simulink model "MSREPrimaryLoop_PlantLevel"  (R2024a)
settings: Solver=VariableStepAuto  StartTime=0.0  StopTime=500000  MaxStep=0.1  RelTol=1e-3
undefined symbols (not defined in the file): a_f, a_g, axialFuelImportance, axialGraphiteImportance, axialPowerFraction, beta, beta_t, bubbleSaturationLevel, bypassRatio, C0, coolantPHXChannelLength, coolantPHXDh, coolantPHXFlowArea, coreCorrectionNominalFlowRate, coreDowncomerArea, coreDowncomerHydraulicDiameter, coreDowncomerLength, coreDowncomerVolume, coreFlowArea, coreFuelVolume, coreInletFlowDistributerArea, coreInletFlowDistributerHydralicDiameter, coreInletFlowDistributerLength, coreInletFlowDistributerVolume, coreLowerPlenumArea, coreLowerPlenumHydraulicDiameter, coreLowerPlenumLength, coreLowerPlenumVolume, coreUpperPlenumArea, coreUpperPlenumLength, coreUpperPlenumVolume, coreVolume, cpGraphite, day, decayScale, decaySSFraction, dissolusionRatio, dMin, dScale, dsmConst, DXeG, externalReactivity, Fiss_factor, fuelChannelHydrualicDiameter, fuelChannelLength, fuelDepositRatio, fuelFraction, fuelGraphiteArea, fuelGraphiteHeatTransferCoefficient, gamma0, gamma1, gamma2, gasExchangeRatio, gasMixingEfficiency, gasPurgeRate, gasStrippingEfficiency, graphiteKDiff, graphiteUnitCellThickness, initialIodineConcentration, InitialXeMolarConcentration ... (+66)
libraries: fl_lib x291, nesl_utility x101, SimscapeFluids_lib x24, simulink x5, slpidlib x1
(part 13 of 13)

== system MSREPrimaryLoop_PlantLevel/Reactor/CoreTH&Inerti/UpperPlenum/XenonCalc/Salt/Subsystem1 ==
  Gas : Inport
  Add1 : Sum  Inputs=+-
  Constant : Constant
  Subsystem : Subsystem  ReferencedSubsystem=GasToAlpha
  1-alpha : Outport
  wires:
  Gas/1 -> Subsystem/1
  Constant/1 -> Add1/1
  Subsystem/1 -> Add1/2
  Add1/1 -> 1-alpha/1

== system MSREPrimaryLoop_PlantLevel/Reactor/Reactivity&PKE/Reactivity&PKE/REACTIVITY/ExternalReactivity/Constatnt ==
  Constant : Constant  Value=0
  y : Outport
  wires:
  Constant/1 -> y/1

== system MSREPrimaryLoop_PlantLevel/Reactor/Reactivity&PKE/Reactivity&PKE/REACTIVITY/ExternalReactivity/Frequency ==
  Sine Wave : Sin  Amplitude=1e-5  Frequency=testFrequency  SampleTime=0.1
  y : Outport
  wires:
  Sine Wave/1 -> y/1

== system MSREPrimaryLoop_PlantLevel/Reactor/Reactivity&PKE/Reactivity&PKE/REACTIVITY/ExternalReactivity/Step ==
  Step : Step  Time=3*day + 1  After=stepReactivity  SampleTime=0
  y : Outport
  wires:
  Step/1 -> y/1

== system MSREPrimaryLoop_PlantLevel/Reactor/Reactivity&PKE/Reactivity&PKE/REACTIVITY/ExternalReactivity/White Noise ==
  Band-Limited White Noise : simulink/Sources/Band-Limited White Noise  Cov=1e-10  Ts=0.1  seed=[23341]
  y : Outport
  wires:
  Band-Limited White Noise/1 -> y/1

== system MSREPrimaryLoop_PlantLevel/Reactor/CoreTH&Inerti/Core/CoreXenonCalc/InterphaseTranfser/Constitutive/Subsystem ==
  note: Include the form loss to averaged frictional factor as a rough estimate.
  PLoss : Inport
  Dh : Inport  Port=2
  ul : Inport  Port=3
  alpha : Inport  Port=4
  Absolute Reference (TL) : fl_lib/Thermal Liquid/Elements/Absolute Reference (TL)
  Constant : Constant  Value=dissolusionRatio
  Constant1 : Constant  Value=dMin
  Constant2 : Constant  Value=dScale
  Constant3 : Constant  Value=dsmConst
  Divide : Product  Inputs=**//
  Gain : Gain  Gain=2/CoreLength
  MATLAB Function1 : MATLAB Function  TreatAsAtomicUnit=on
  MATLAB Function2 : MATLAB Function  TreatAsAtomicUnit=on
  Math Function : Math  Operator=square
  PS-Simulink Converter : nesl_utility/PS-Simulink Converter  PhysicalDomain=network_engine_domain  SubClassName=ps_output  LeftPortType=input  RightPortType=output  PseudoPeriodic=off  Frequencies=[]  VectorFormat=1-D array  Unit=inherit  AffineConversion=off
  PS-Simulink Converter1 : nesl_utility/PS-Simulink Converter  PhysicalDomain=network_engine_domain  SubClassName=ps_output  LeftPortType=input  RightPortType=output  PseudoPeriodic=off  Frequencies=[]  VectorFormat=1-D array  Unit=inherit  AffineConversion=off
  Pressure & Temperature Sensor (TL) : fl_lib/Thermal Liquid/Sensors/Pressure & Temperature Sensor (TL)  reference=foundation.enum.MeasurementReference.difference  pressure=true  pressure_spec=foundation.enum.PressureMeasementSpec.Absolute  temperature=true
      settings: InternalSimscapePortConfiguration="{\"Bottom\":[{\"id\":\"T\",\"label\":\"T\",\"type\":\"output\"}],\"Left\":[{\"id\":\"A\",\"label\":\"A\",\"type\":\"foundation.thermal_liquid.thermal_liquid\"}],\"Right\":[{\"id\":\"B\",\"label\":\"B\",\"type\":\"foundation.thermal_liquid.thermal_liquid\"},{\"id\":\"P\",\"label\":\"P\",\"type\":\"output\"}],\"Top\":[]}"
  Simscape Component : SimscapeComponentBlock  SourceFile=TL_FullSensor  ComponentPath=TL_FullSensor  ComponentVariants="[\"TL_FullSensor\"]"  ComponentVariantNames="[\"TL_FullSensor\"]"  ClassName=TL_FullSensor  SchemaVersion=1
      settings: CopyFcn=simscape.engine.sli.internal.componentblockcallback(gcbh,'COPY')  PreCopyFcn=simscape.engine.sli.internal.componentblockcallback(gcbh,'PRECOPY')  PreDeleteFcn=simscape.engine.sli.internal.componentblockcallback(gcbh,'PREDELETE')  InternalSimscapePortConfiguration="{\"Bottom\":[],\"Left\":[{\"id\":\"A\",\"label\":\"A\",\"type\":\"foundation.thermal_liquid.thermal_liquid\"}],\"Right\":[{\"id\":\"U\",\"label\":\"u\",\"type\":\"output\"},{\"id\":\"RHO\",\"label\":\"rho\",\"type\":\"output\"},{\"id\":\"CP\",\"label\":\"cp\",\"type\":\"output\"},{\"id\":\"NU\",\"label\":\"nu\",\"type\":\"output\"}],\"Top\":[]}"
      mask Type: Thermodynamic Properties Sensor (TL)
      mask Display: color('red');plot([0 1 1 0 0],[0 0 1 1 0]);plot([0.7,1],[1,0.7]);plot(-2,-1.75);plot(3, 1);disp('\n.ssc\nUnresolved')
  Terminator1 : Terminator
  Ref : PMIOPort  Side=Right
  f_Combined : Outport
  dsm : Outport  Port=2
  wires:
  Dh/1 -> Divide/2, MATLAB Function1/2(D)
  MATLAB Function2/1(sigma) -> MATLAB Function1/5(sigma)
  PS-Simulink Converter1/1 -> MATLAB Function2/1(T)
  ul/1 -> Math Function/1, MATLAB Function1/3(jl)
  PS-Simulink Converter/1 -> Divide/4, MATLAB Function1/4(rhol)
  PLoss/1 -> Gain/1
  Divide/1 -> f_Combined/1, MATLAB Function1/1(f)
  Gain/1 -> Divide/1
  Math Function/1 -> Divide/3
  alpha/1 -> MATLAB Function1/6(alpha)
  Constant/1 -> MATLAB Function1/7(alphaDissolve)
  Constant1/1 -> MATLAB Function1/8(dMin)
  Constant2/1 -> MATLAB Function1/9(scale)
  Constant3/1 -> dsm/1
  MATLAB Function1/1(dsm) -> Terminator1/1
  connections:
  Simscape Component/RConn2 -- PS-Simulink Converter/LConn1
  Simscape Component/LConn1 -- Pressure & Temperature Sensor (TL)/LConn1 -- Ref/RConn1
  Pressure & Temperature Sensor (TL)/RConn3 -- PS-Simulink Converter1/LConn1
  Pressure & Temperature Sensor (TL)/RConn1 -- Absolute Reference (TL)/LConn1

== system MSREPrimaryLoop_PlantLevel/Reactor/CoreTH&Inerti/Core/CoreXenonCalc/InterphaseTranfser/GraphiteInterchangeModel/GasDiffusivityScale ==
  T : Inport
  Constant : Constant  Value=1.5
  Divide : Product  Inputs=*/
  Divide1 : Product  Inputs=*/
  PReff : Constant  Value=1.013e5
  Power : Math  Operator=pow
  Product : Product  Inputs=3
  TRef : Constant  Value=900
  XeReferenceDiff : Constant  Value=DXeG
  DiffGas : Outport
  wires:
  T/1 -> Divide/1
  TRef/1 -> Divide/2
  Divide/1 -> Power/1
  Constant/1 -> Power/2
  PReff/1 -> Divide1/1
  [coreAveragePressure] -> Divide1/2
  Power/1 -> Product/1
  Divide1/1 -> Product/2
  XeReferenceDiff/1 -> Product/3
  Product/1 -> DiffGas/1

== system MSREPrimaryLoop_PlantLevel/Reactor/CoreTH&Inerti/Core/Subsystem2/Subsystem2/If Action Subsystem/SolubilityModificationEqual ==
  note: The idea is that when the dissolved gas comes back out, it is at the same salt concentration, assuming the nucleation process is fast, and it absorbed all xenon at the nucleation site but diffusion is not yet to kick in. As for the absorption into the old bubble, the saturation may be closer to 0, but never the less, the saturation level is already close to zero.
  XeIn : Inport
  CoreGas : Inport  Port=2
  DissolvedGas : Inport  Port=3
  Add : Sum
  Add1 : Sum
  AddedBackGas : Sum
  Constant : Constant
  Demux : Demux  Outputs=2
  Divide : Product  Inputs=**/
  Divide1 : Product  Inputs=*/
  Mux : Mux  Inputs=2
  XeOut : Outport
  GasOut : Outport  Port=2
  wires:
  CoreGas/1 -> AddedBackGas/1
  AddedBackGas/1 -> GasOut/1
  XeIn/1 -> Demux/1
  Mux/1 -> XeOut/1
  Constant/1 -> Add/2
  Add/1 -> Divide1/2, Divide/3
  Demux/1 -> Divide/1, Divide1/1
  Demux/2 -> Add1/1
  Divide/1 -> Add1/2
  Add1/1 -> Mux/2
  Divide1/1 -> Mux/1
  DissolvedGas/1 -> Add/1, Divide/2, AddedBackGas/2

== system MSREPrimaryLoop_PlantLevel/Reactor/CoreTH&Inerti/Core/Subsystem2/Subsystem2/If Action Subsystem1/SolubilityModificationPrescribed ==
  note: The idea is that when the dissolved gas comes back out, it is saturated with xenon because of the super efficiency removal of micro bubbles. The gain factor is used to adjust the concentration of the bubbles to less than saturation.
  XeIn : Inport
  CoreGas : Inport  Port=2
  DissolvedGas : Inport  Port=3
  Temperature : Inport  Port=4
  Add : Sum
  Add1 : Sum
  AddedBackGas : Sum
  Constant : Constant
  Demux : Demux  Outputs=2
  Divide : Product  Inputs=**/
  Divide1 : Product  Inputs=*/
  Divide2 : Product  Inputs=*/
  Gain : Gain  Gain=bubbleSaturationLevel
  KScale : Subsystem  ReferencedSubsystem=KScale
  Mux : Mux  Inputs=2
  XeOut : Outport
  GasOut : Outport  Port=2
  wires:
  CoreGas/1 -> AddedBackGas/1
  DissolvedGas/1 -> Divide2/1, AddedBackGas/2
  AddedBackGas/1 -> GasOut/1
  XeIn/1 -> Demux/1
  Mux/1 -> XeOut/1
  Temperature/1 -> KScale/1
  KScale/1 -> Divide2/2
  Constant/1 -> Add/2
  Divide2/1 -> Gain/1
  Add/1 -> Divide1/2, Divide/3
  Demux/1 -> Divide/1, Divide1/1
  Demux/2 -> Add1/1
  Divide/1 -> Add1/2
  Add1/1 -> Mux/2
  Divide1/1 -> Mux/1
  Gain/1 -> Add/1, Divide/2

== matlab function MSREPrimaryLoop_PlantLevel/Reactor/CoreTH&Inerti/DownComer/XenonCalc/InterphaseTranfser/Transfer Term ==
  settings: updateMethod=DISCRETE
  data: GxS input; GxG input; volRate output; alpha input; ul input; ug input; K input; dsm input; k input
function volRate = Interpahse(GxS, GxG, alpha, ul, ug, K, dsm, k)

%Using GxS and GxG as variable is good for implementation to incorporate
%the initialization without divergence
volRate = 6*k/dsm*(K*GxG/ug - alpha/(1-alpha)*GxS/ul);

== matlab function MSREPrimaryLoop_PlantLevel/pipePHXToReactor/XenonCalc/InterphaseTranfser/Transfer Term ==
  settings: updateMethod=DISCRETE
  data: GxS input; GxG input; volRate output; alpha input; ul input; ug input; K input; dsm input; k input
function volRate = Interpahse(GxS, GxG, alpha, ul, ug, K, dsm, k)

%Using GxS and GxG as variable is good for implementation to incorporate
%the initialization without divergence
volRate = 6*k/dsm*(K*GxG/ug - alpha/(1-alpha)*GxS/ul);

== matlab function MSREPrimaryLoop_PlantLevel/PHX Physical/XenonCalc/InterphaseTranfser/Transfer Term ==
  settings: updateMethod=DISCRETE
  data: GxS input; GxG input; volRate output; alpha input; ul input; ug input; K input; dsm input; k input
function volRate = Interpahse(GxS, GxG, alpha, ul, ug, K, dsm, k)

%Using GxS and GxG as variable is good for implementation to incorporate
%the initialization without divergence
volRate = 6*k/dsm*(K*GxG/ug - alpha/(1-alpha)*GxS/ul);

== matlab function MSREPrimaryLoop_PlantLevel/pipePumpToPHX/XenonCalc/InterphaseTranfser/Transfer Term ==
  settings: updateMethod=DISCRETE
  data: GxS input; GxG input; volRate output; alpha input; ul input; ug input; K input; dsm input; k input
function volRate = Interpahse(GxS, GxG, alpha, ul, ug, K, dsm, k)

%Using GxS and GxG as variable is good for implementation to incorporate
%the initialization without divergence
volRate = 6*k/dsm*(K*GxG/ug - alpha/(1-alpha)*GxS/ul);

== matlab function MSREPrimaryLoop_PlantLevel/Pump MSRE/Pump Bowl/Salt Space/XenonCalcBowl/InterphaseTranfser/Transfer Term ==
  settings: updateMethod=DISCRETE
  data: CxS input; CxG input; volRate output; alpha input; K input; dsm input; k input
function volRate = InterpahseSimple(CxS, CxG, alpha, K, dsm, k)

%Using GxS and GxG as variable is good for implementation to incorporate
%the initialization without divergence
volRate = 6*k*alpha/dsm*(K*CxG - CxS);

== matlab function MSREPrimaryLoop_PlantLevel/Reactor/CoreTH&Inerti/UpperPlenum/XenonCalc/InterphaseTranfser/Transfer Term ==
  settings: updateMethod=DISCRETE
  data: GxS input; GxG input; volRate output; alpha input; ul input; ug input; K input; dsm input; k input
function volRate = Interpahse(GxS, GxG, alpha, ul, ug, K, dsm, k)

%Using GxS and GxG as variable is good for implementation to incorporate
%the initialization without divergence
volRate = 6*k/dsm*(K*GxG/ug - alpha/(1-alpha)*GxS/ul);

== matlab function MSREPrimaryLoop_PlantLevel/Reactor/CoreTH&Inerti/Inlet Distribution/XenonCalc/InterphaseTranfser/Transfer Term ==
  settings: updateMethod=DISCRETE
  data: GxS input; GxG input; volRate output; alpha input; ul input; ug input; K input; dsm input; k input
function volRate = Interpahse(GxS, GxG, alpha, ul, ug, K, dsm, k)

%Using GxS and GxG as variable is good for implementation to incorporate
%the initialization without divergence
volRate = 6*k/dsm*(K*GxG/ug - alpha/(1-alpha)*GxS/ul);

== matlab function MSREPrimaryLoop_PlantLevel/Reactor/CoreTH&Inerti/LowerPlenum/XenonCalc/InterphaseTranfser/Transfer Term ==
  settings: updateMethod=DISCRETE
  data: GxS input; GxG input; volRate output; alpha input; ul input; ug input; K input; dsm input; k input
function volRate = Interpahse(GxS, GxG, alpha, ul, ug, K, dsm, k)

%Using GxS and GxG as variable is good for implementation to incorporate
%the initialization without divergence
volRate = 6*k/dsm*(K*GxG/ug - alpha/(1-alpha)*GxS/ul);

== matlab function MSREPrimaryLoop_PlantLevel/Reactor/CoreTH&Inerti/Core/CoreXenonCalc/InterphaseTranfser/Transfer Term ==
  settings: updateMethod=DISCRETE
  data: GxS input; GxG input; volRate output; alpha input; ul input; ug input; K input; dsm input; k input
function volRate = Interpahse(GxS, GxG, alpha, ul, ug, K, dsm, k)

%Using GxS and GxG as variable is good for implementation to incorporate
%the initialization without divergence
volRate = 6*k/dsm*(K*GxG/ug - alpha/(1-alpha)*GxS/ul);

== matlab function MSREPrimaryLoop_PlantLevel/Reactor/CoreTH&Inerti/Core/CoreXenonCalc/InterphaseTranfser/GraphiteInterchangeModel/GraphiteDiffusion ==
  settings: updateMethod=DISCRETE
  data: tnp1 input; CXef input; CXeg input; phi input; fluxSalt output; fluxGas output; alpha input; xe_pvolave_conc output; K input; Df input; Dg input; d input; shapeFactor input; C_face output; ul input; graphiteKD input
function [fluxSalt, fluxGas, xe_pvolave_conc, C_face] = xeMSREGraphite(tnp1, CXef,CXeg, phi, alpha, K, Df, Dg, d, shapeFactor, ul,graphiteKD)
%Solve diffusion into the graphite
    persistent tn
    persistent xegrid
    persistent rgrid
    persistent A
    persistent g

    porosity = 0.1;
    Dh = 0.0159; %MSRE unit flow cell.

    %It is expected that the regime is in laminar flow, the Kedl model used
    %a weird engineering correlation and gives a much larger
    %value for k. 
    kl = 3.66*Df/Dh;
    %Two layer model for overall mass transfer
    Rl = 1/kl;
    Rd = 0.2e-6/Df/sqrt(porosity);
    k = 1/(Rl + Rd);
  

    XeDecayConstant = 2.0916e-05;
    sigma_xe135 = 2.7e-18;

    R = 0.0277;
    dr = R/30;
    %Dk = 1.45e-8;
    Dk = graphiteKD; %A complicated topic, best left as a parameter.  See document.
    %Deff = 1.32e-8; %Taken from ORNL-4148 p35
    Deff = Dk*Dg/(Dk+Dg);
    
    ug = ul + 1e-3;
    dstar = sqrt(Dg*d/ug);
    
    %Used to adjust the shape factor, with k_g_eff = Dg/d * factor
  
   
    shapeFactor = max(shapeFactor*exp(-5e-4/d)*porosity,4*k*sqrt(d/Dg/ug));
  
    Dg = shapeFactor * Dg;


    %The diffusion term should not be dependent upto D/d. Rather, it's
    %porosity*sqrt(D*u/d), here we define dstar = sqrt(Dd/u) so that we
    %don't have to modify the code
    
    %could make a drift velocity formulation, ignored for now
    
    d = dstar;

    %Initialization of the persistent variables if the function is first
    %time being used
    if isempty(tn)
        tn = 0;
    end
    if isempty(rgrid)
        rgrid = linspace(0+dr/2,R-dr/2,30)';
    end
    if isempty(xegrid)
        xegrid = zeros(size(rgrid));
    end

    if isempty(g)
        g = zeros(size(rgrid));
        g(end) = (Deff/dr^2+Deff/2/dr)*2*k*dr/(2*porosity*Deff+K*k*dr)*CXef;
    end
    
    dt = tnp1 - tn;
    tn = tnp1;

    if dt <eps
        %Initialize to steady state condition if tnp1<=tn.
        tn = 0;
        %Use phi0 for initialization flux. This feels not always
        %appropriate
        phi0 = 0;
        phi = phi0;
        termp1 = Deff/dr^2*ones(length(rgrid)-1,1)+Deff/2/dr./rgrid(1:end-1);
        termm1 = Deff/dr^2*ones(length(rgrid)-1,1)-Deff/2/dr./rgrid(2:end);
        termdiag = -(2*Deff/dr^2+XeDecayConstant+phi*sigma_xe135)*ones(size(rgrid));
        lumpedDemominator = Dg*alpha*dr + 2*Deff*d*porosity + K*d*dr*k - K*alpha*d*dr*k;
        frontFactorCn = (2*Deff*d*porosity - Dg*alpha*dr - K*d*dr*k + K*alpha*d*dr*k)/lumpedDemominator;
        %reference no alpha, cn , (2*porosity*Deff-K*k*dr)/(2*porosity*Deff+K*k*dr)
        termdiag(end) = termdiag(end) + (Deff/dr^2+Deff/2/dr./rgrid(end))*frontFactorCn;
        A = diag(termp1,1)+diag(termm1,-1)+diag(termdiag);
        %reference no alpha, g, 2*k*dr/(2*porosity*Deff+K*k*dr)*CXef
        frontFactorBc = (2*Dg*alpha*CXeg*dr + 2*CXef*d*dr*k - 2*alpha*CXef*d*dr*k)/lumpedDemominator;
        g(end) = (Deff/dr^2+Deff/2/dr./rgrid(end))*frontFactorBc;

        xegrid = -A\g;
        %Reference no alpha, (2*porosity*Deff-K*k*dr)/(2*porosity*Deff+K*k*dr)*xegrid(end) + 2*k*dr/(2*porosity*Deff+K*k*dr)*CXef
        C_ghost = frontFactorBc + frontFactorCn*xegrid(end);
        C_face = (xegrid(end) + C_ghost)/2;

        fluxSalt = k*(K*C_face-CXef)*(1-alpha);
        fluxGas = alpha*Dg/d*(C_face-CXeg);
        
        %Calculate phase volume averaged concentration
        xe_pvolave_conc = sum(((rgrid+dr/2).^2-(rgrid-dr/2).^2).*xegrid)/R^2;

   
        

    else
        %Backward Euler time advancement scheme
        I = diag(ones(size(rgrid)));
        
        %Update time-dependent matrix
        termp1 = Deff/dr^2*ones(length(rgrid)-1,1)+Deff/2/dr./rgrid(1:end-1);
        termm1 = Deff/dr^2*ones(length(rgrid)-1,1)-Deff/2/dr./rgrid(2:end);
        termdiag = -(2*Deff/dr^2+XeDecayConstant+phi*sigma_xe135)*ones(size(rgrid));
        lumpedDemominator = Dg*alpha*dr + 2*Deff*d*porosity + K*d*dr*k - K*alpha*d*dr*k;
        frontFactorCn = (2*Deff*d*porosity - Dg*alpha*dr - K*d*dr*k + K*alpha*d*dr*k)/lumpedDemominator;
        %reference no alpha, cn , (2*porosity*Deff-K*k*dr)/(2*porosity*Deff+K*k*dr)
        termdiag(end) = termdiag(end) + (Deff/dr^2+Deff/2/dr./rgrid(end))*frontFactorCn;
        A = diag(termp1,1)+diag(termm1,-1)+diag(termdiag);
        %reference no alpha, g, 2*k*dr/(2*porosity*Deff+K*k*dr)*CXef
        frontFactorBc = (2*Dg*alpha*CXeg*dr + 2*CXef*d*dr*k - 2*alpha*CXef*d*dr*k)/lumpedDemominator;
        g(end) = (Deff/dr^2+Deff/2/dr./rgrid(end))*frontFactorBc;
        
        %Solve for new xenon concentration profile
        xegrid = (I-A*dt)\(g*dt+xegrid);
        
        %Calculate xenon flux in at the boundary
        C_ghost = frontFactorBc + frontFactorCn*xegrid(end);
        C_face = (xegrid(end) + C_ghost)/2;

        fluxSalt = k*(K*C_face-CXef)*(1-alpha);
        fluxGas = alpha*Dg/d*(C_face-CXeg);
        
        %Calculate phase volume averaged concentration
        xe_pvolave_conc = sum(((rgrid+dr/2).^2-(rgrid-dr/2).^2).*xegrid)/R^2;

    end

== matlab function MSREPrimaryLoop_PlantLevel/Pump MSRE/Pump/PumpIdeal/XenonCalcPump/InterphaseTranfser/Transfer Term ==
  settings: updateMethod=DISCRETE
  data: CxS input; CxG input; volRate output; alpha input; K input; dsm input; k input
function volRate = InterpahseSimple(CxS, CxG, alpha, K, dsm, k)

%Using GxS and GxG as variable is good for implementation to incorporate
%the initialization without divergence
volRate = 6*k*alpha/dsm*(K*CxG - CxS);

== matlab function MSREPrimaryLoop_PlantLevel/Reactor/CoreTH&Inerti/Core/CoreXenonCalc/InterphaseTranfser/Constitutive/Subsystem/MATLAB Function1 ==
  settings: updateMethod=DISCRETE
  data: f input; D input; jl input; rhol input; sigma input; dsm output; alpha input; alphaDissolve input; dMin input; scale input
function dsm = dsmTurbulent(f,D,jl,rhol,sigma,alpha,alphaDissolve,dMin,scale)

%alphaDissolve = max(eps,alphaDissolve);
dissipation = jl^3/2/D*abs(f);
dsm = scale*0.725/(rhol/sigma)^0.6/dissipation^0.4;
x = -atanh(2*dMin/dsm-1);
%dsm = max(dsm*(0.5 + 0.5*tanh(alpha*250-x))*(alpha./(alphaDissolve+alpha)).^(1/3),1e-5);
dsm = max(dsm*(0.5 + 0.5*tanh(alpha*100-x))*(alpha./(alphaDissolve+alpha)).^(1/3),1e-5);
%dsm = min(dsm,dMin*(1+alpha.^2))
dsm = min(dsm,D);

end

== matlab function MSREPrimaryLoop_PlantLevel/Reactor/CoreTH&Inerti/Core/CoreXenonCalc/InterphaseTranfser/Constitutive/Subsystem/MATLAB Function2 ==
  data: T input; sigma output
function sigma = sigmaEquation(T)

T = T-273.15;
sigma = (235.5-0.09*T)*0.001; %Source from solubility in FLiBe by WATSON et al.

end

== matlab function MSREPrimaryLoop_PlantLevel/pipeReactorToPump/XenonCalc/InterphaseTranfser/Transfer Term ==
  settings: updateMethod=DISCRETE
  data: GxS input; GxG input; volRate output; alpha input; ul input; ug input; K input; dsm input; k input
function volRate = Interpahse(GxS, GxG, alpha, ul, ug, K, dsm, k)

%Using GxS and GxG as variable is good for implementation to incorporate
%the initialization without divergence
volRate = 6*k/dsm*(K*GxG/ug - alpha/(1-alpha)*GxS/ul);
